simulink model "AN_Simulink_Model_v1_fil"  (R2019b)
settings: Solver=VariableStepAuto  StartTime=0.0  StopTime=testtime  RelTol=1e-3
InitFcn:
  | AN_InitFcn_Callback
StopFcn:
  | AN_StopFcn_Callback
undefined symbols (not defined in the file or in its folder): tdres
libraries: hdlmdlgenlib x193, simulink x4, fillib x1, dspsrcs4 x1
(part 5 of 6)

== system AN_Simulink_Model_v1_fil/Auditory Nerve Model/C2 Wideband Filter/Calculate C2filterout/Abs ==
  In1 : Inport
  Abs : Abs  SampleTime=2.08333333333333e-05  OutDataTypeStr=single
  Out1 : Outport
  wires:
  Abs/1 -> Out1/1
  In1/1 -> Abs/1

== system AN_Simulink_Model_v1_fil/Auditory Nerve Model/C2 Wideband Filter/Calculate C2filterout/Divide ==
  In1 : Inport
  In2 : Inport  Port=2
  Divide : Product  Inputs=*/  OutDataTypeStr=single  SampleTime=2.08333333333333e-05  SaturateOnIntegerOverflow=on  RndMeth=Zero
  Out1 : Outport
  wires:
  Divide/1 -> Out1/1
  In2/1 -> Divide/2
  In1/1 -> Divide/1

== system AN_Simulink_Model_v1_fil/Auditory Nerve Model/C2 Wideband Filter/Calculate C2filterout/Divide1 ==
  In1 : Inport
  In2 : Inport  Port=2
  Divide1 : Product  Inputs=*/  OutDataTypeStr=single  SampleTime=2.08333333333333e-05  SaturateOnIntegerOverflow=on  RndMeth=Zero
  Out1 : Outport
  wires:
  Divide1/1 -> Out1/1
  In2/1 -> Divide1/2
  In1/1 -> Divide1/1

== system AN_Simulink_Model_v1_fil/Auditory Nerve Model/C2 Wideband Filter/Calculate C2filterout/Product ==
  In1 : Inport
  In2 : Inport  Port=2
  Product : Product  Inputs=**  OutDataTypeStr=single  SampleTime=2.08333333333333e-05
  Out1 : Outport
  wires:
  Product/1 -> Out1/1
  In2/1 -> Product/2
  In1/1 -> Product/1

== system AN_Simulink_Model_v1_fil/Auditory Nerve Model/C2 Wideband Filter/Calculate C2filterout/Product1 ==
  In1 : Inport
  In2 : Inport  Port=2
  Product1 : Product  Inputs=**  OutDataTypeStr=single  SampleTime=2.08333333333333e-05
  Out1 : Outport
  wires:
  Product1/1 -> Out1/1
  In2/1 -> Product1/2
  In1/1 -> Product1/1

== system AN_Simulink_Model_v1_fil/Auditory Nerve Model/C2 Wideband Filter/Calculate C2filterout/Product2 ==
  In1 : Inport
  In2 : Inport  Port=2
  Product2 : Product  Inputs=**  OutDataTypeStr=single  SampleTime=2.08333333333333e-05
  Out1 : Outport
  wires:
  Product2/1 -> Out1/1
  In2/1 -> Product2/2
  In1/1 -> Product2/1

== system AN_Simulink_Model_v1_fil/Auditory Nerve Model/CP Wideband Gammatone Filter/Calculate wbout/Divide ==
  In1 : Inport
  In2 : Inport  Port=2
  Divide : Product  Inputs=*/  OutDataTypeStr=single  SampleTime=2.08333333333333e-05  SaturateOnIntegerOverflow=on  RndMeth=Zero
  Out1 : Outport
  wires:
  Divide/1 -> Out1/1
  In2/1 -> Divide/2
  In1/1 -> Divide/1

== system AN_Simulink_Model_v1_fil/Auditory Nerve Model/CP Wideband Gammatone Filter/Calculate wbout/Gain ==
  In1 : Inport
  In2 : Inport  Port=2
  Gain : Product  Inputs=**  OutDataTypeStr=single  SampleTime=2.08333333333333e-05
  Out1 : Outport
  wires:
  Gain/1 -> Out1/1
  In2/1 -> Gain/2
  In1/1 -> Gain/1

== system AN_Simulink_Model_v1_fil/Auditory Nerve Model/CP Wideband Gammatone Filter/Calculate wbout/MinMax_stage1_compare ==
  In1 : Inport
  In2 : Inport  Port=2
  MinMax_stage1_compare : RelationalOperator  Operator=<  OutDataTypeStr=boolean  SampleTime=2.08333333333333e-05  RndMeth=Nearest  InputSameDT=on
  Out1 : Outport
  wires:
  MinMax_stage1_compare/1 -> Out1/1
  In2/1 -> MinMax_stage1_compare/2
  In1/1 -> MinMax_stage1_compare/1

== system AN_Simulink_Model_v1_fil/Auditory Nerve Model/CP Wideband Gammatone Filter/Calculate wbout/Pow ==
  In1 : Inport
  In2 : Inport  Port=2
  Pow : Math  Operator=pow  SampleTime=2.08333333333333e-05  SaturateOnIntegerOverflow=on
  Out1 : Outport
  wires:
  Pow/1 -> Out1/1
  In2/1 -> Pow/2
  In1/1 -> Pow/1

== system AN_Simulink_Model_v1_fil/Auditory Nerve Model/CP Wideband Gammatone Filter/Calculate wbout/Product ==
  In1 : Inport
  In2 : Inport  Port=2
  Product : Product  Inputs=**  OutDataTypeStr=single  SampleTime=2.08333333333333e-05
  Out1 : Outport
  wires:
  Product/1 -> Out1/1
  In2/1 -> Product/2
  In1/1 -> Product/1

== system AN_Simulink_Model_v1_fil/Auditory Nerve Model/CP Wideband Gammatone Filter/Calculate wbout/Product1 ==
  In1 : Inport
  In2 : Inport  Port=2
  Product1 : Product  Inputs=**  OutDataTypeStr=single  SampleTime=2.08333333333333e-05
  Out1 : Outport
  wires:
  Product1/1 -> Out1/1
  In2/1 -> Product1/2
  In1/1 -> Product1/1

== system AN_Simulink_Model_v1_fil/Auditory Nerve Model/CP Wideband Gammatone Filter/MATLAB Function1/adder ==
  In1 : Inport
  In2 : Inport  Port=2
  adder : Sum  OutDataTypeStr=single  SampleTime=2.08333333333333e-05  SaturateOnIntegerOverflow=on  InputSameDT=on
  Out1 : Outport
  wires:
  adder/1 -> Out1/1
  In2/1 -> adder/2
  In1/1 -> adder/1

== system AN_Simulink_Model_v1_fil/Auditory Nerve Model/CP Wideband Gammatone Filter/MATLAB Function1/relop ==
  In1 : Inport
  In2 : Inport  Port=2
  relop : RelationalOperator  Operator=<=  OutDataTypeStr=boolean  SampleTime=2.08333333333333e-05  RndMeth=Nearest
  Out1 : Outport
  wires:
  relop/1 -> Out1/1
  In2/1 -> relop/2
  In1/1 -> relop/1

== system AN_Simulink_Model_v1_fil/Auditory Nerve Model/CP Wideband Gammatone Filter/MATLAB Function1/subtract ==
  In1 : Inport
  In2 : Inport  Port=2
  subtract : Sum  Inputs=+-  OutDataTypeStr=single  SampleTime=2.08333333333333e-05  SaturateOnIntegerOverflow=on  InputSameDT=on
  Out1 : Outport
  wires:
  subtract/1 -> Out1/1
  In2/1 -> subtract/2
  In1/1 -> subtract/1

== system AN_Simulink_Model_v1_fil/Auditory Nerve Model/CP Wideband Gammatone Filter/Third Order IIR Filter/Add ==
  In1 : Inport
  In2 : Inport  Port=2
  Add : Sum  OutDataTypeStr=single  SampleTime=2.08333333333333e-05  SaturateOnIntegerOverflow=on  InputSameDT=on
  Out1 : Outport
  wires:
  Add/1 -> Out1/1
  In2/1 -> Add/2
  In1/1 -> Add/1

== system AN_Simulink_Model_v1_fil/Auditory Nerve Model/CP Wideband Gammatone Filter/Third Order IIR Filter/Divide ==
  In1 : Inport
  In2 : Inport  Port=2
  Divide : Product  Inputs=*/  OutDataTypeStr=single  SampleTime=2.08333333333333e-05  SaturateOnIntegerOverflow=on  RndMeth=Zero
  Out1 : Outport
  wires:
  Divide/1 -> Out1/1
  In2/1 -> Divide/2
  In1/1 -> Divide/1

== system AN_Simulink_Model_v1_fil/Auditory Nerve Model/CP Wideband Gammatone Filter/Third Order IIR Filter/Divide1 ==
  In1 : Inport
  In2 : Inport  Port=2
  Divide1 : Product  Inputs=*/  OutDataTypeStr=single  SampleTime=2.08333333333333e-05  SaturateOnIntegerOverflow=on  RndMeth=Zero
  Out1 : Outport
  wires:
  Divide1/1 -> Out1/1
  In2/1 -> Divide1/2
  In1/1 -> Divide1/1

== system AN_Simulink_Model_v1_fil/Auditory Nerve Model/CP Wideband Gammatone Filter/Third Order IIR Filter/Divide2 ==
  In1 : Inport
  In2 : Inport  Port=2
  Divide2 : Product  Inputs=*/  OutDataTypeStr=single  SampleTime=2.08333333333333e-05  SaturateOnIntegerOverflow=on  RndMeth=Zero
  Out1 : Outport
  wires:
  Divide2/1 -> Out1/1
  In2/1 -> Divide2/2
  In1/1 -> Divide2/1

== system AN_Simulink_Model_v1_fil/Auditory Nerve Model/CP Wideband Gammatone Filter/Third Order IIR Filter/Product2 ==
  In1 : Inport
  In2 : Inport  Port=2
  Product2 : Product  Inputs=**  OutDataTypeStr=single  SampleTime=2.08333333333333e-05
  Out1 : Outport
  wires:
  Product2/1 -> Out1/1
  In2/1 -> Product2/2
  In1/1 -> Product2/1

== system AN_Simulink_Model_v1_fil/Auditory Nerve Model/CP Wideband Gammatone Filter/Third Order IIR Filter/Product21 ==
  In1 : Inport
  In2 : Inport  Port=2
  Product21 : Product  Inputs=**  OutDataTypeStr=single  SampleTime=2.08333333333333e-05
  Out1 : Outport
  wires:
  Product21/1 -> Out1/1
  In2/1 -> Product21/2
  In1/1 -> Product21/1

== system AN_Simulink_Model_v1_fil/Auditory Nerve Model/CP Wideband Gammatone Filter/Third Order IIR Filter/Product3_to_gain ==
  In1 : Inport
  Product3_to_gain : Gain  Gain=single(2)
  Out1 : Outport
  wires:
  Product3_to_gain/1 -> Out1/1
  In1/1 -> Product3_to_gain/1

== system AN_Simulink_Model_v1_fil/Auditory Nerve Model/CP Wideband Gammatone Filter/Third Order IIR Filter/Product4 ==
  In1 : Inport
  In2 : Inport  Port=2
  Product4 : Product  Inputs=**  OutDataTypeStr=single  SampleTime=2.08333333333333e-05
  Out1 : Outport
  wires:
  Product4/1 -> Out1/1
  In2/1 -> Product4/2
  In1/1 -> Product4/1

== system AN_Simulink_Model_v1_fil/Auditory Nerve Model/CP Wideband Gammatone Filter/Third Order IIR Filter/Product41 ==
  In1 : Inport
  In2 : Inport  Port=2
  Product41 : Product  Inputs=**  OutDataTypeStr=single  SampleTime=2.08333333333333e-05
  Out1 : Outport
  wires:
  Product41/1 -> Out1/1
  In2/1 -> Product41/2
  In1/1 -> Product41/1

== system AN_Simulink_Model_v1_fil/Auditory Nerve Model/CP Wideband Gammatone Filter/Third Order IIR Filter/Product5 ==
  In1 : Inport
  In2 : Inport  Port=2
  Product5 : Product  Inputs=**  OutDataTypeStr=single  SampleTime=2.08333333333333e-05
  Out1 : Outport
  wires:
  Product5/1 -> Out1/1
  In2/1 -> Product5/2
  In1/1 -> Product5/1

== system AN_Simulink_Model_v1_fil/Auditory Nerve Model/CP Wideband Gammatone Filter/Third Order IIR Filter/Product6 ==
  In1 : Inport
  In2 : Inport  Port=2
  Product6 : Product  Inputs=**  OutDataTypeStr=single  SampleTime=2.08333333333333e-05
  Out1 : Outport
  wires:
  Product6/1 -> Out1/1
  In2/1 -> Product6/2
  In1/1 -> Product6/1

== system AN_Simulink_Model_v1_fil/Auditory Nerve Model/CP Wideband Gammatone Filter/Third Order IIR Filter/Product61 ==
  In1 : Inport
  In2 : Inport  Port=2
  Product61 : Product  Inputs=**  OutDataTypeStr=single  SampleTime=2.08333333333333e-05
  Out1 : Outport
  wires:
  Product61/1 -> Out1/1
  In2/1 -> Product61/2
  In1/1 -> Product61/1

== system AN_Simulink_Model_v1_fil/Auditory Nerve Model/CP Wideband Gammatone Filter/Third Order IIR Filter/Product7 ==
  In1 : Inport
  In2 : Inport  Port=2
  Product7 : Product  Inputs=**  OutDataTypeStr=single  SampleTime=2.08333333333333e-05
  Out1 : Outport
  wires:
  Product7/1 -> Out1/1
  In2/1 -> Product7/2
  In1/1 -> Product7/1

== system AN_Simulink_Model_v1_fil/Auditory Nerve Model/CP Wideband Gammatone Filter/Third Order IIR Filter/Product71 ==
  In1 : Inport
  In2 : Inport  Port=2
  Product71 : Product  Inputs=**  OutDataTypeStr=single  SampleTime=2.08333333333333e-05
  Out1 : Outport
  wires:
  Product71/1 -> Out1/1
  In2/1 -> Product71/2
  In1/1 -> Product71/1

== system AN_Simulink_Model_v1_fil/Auditory Nerve Model/CP Wideband Gammatone Filter/Third Order IIR Filter/Product8 ==
  In1 : Inport
  In2 : Inport  Port=2
  Product8 : Product  Inputs=**  OutDataTypeStr=single  SampleTime=2.08333333333333e-05
  Out1 : Outport
  wires:
  Product8/1 -> Out1/1
  In2/1 -> Product8/2
  In1/1 -> Product8/1

== system AN_Simulink_Model_v1_fil/Auditory Nerve Model/CP Wideband Gammatone Filter/Third Order IIR Filter/Product81 ==
  In1 : Inport
  In2 : Inport  Port=2
  Product81 : Product  Inputs=**  OutDataTypeStr=single  SampleTime=2.08333333333333e-05
  Out1 : Outport
  wires:
  Product81/1 -> Out1/1
  In2/1 -> Product81/2
  In1/1 -> Product81/1

== system AN_Simulink_Model_v1_fil/Auditory Nerve Model/CP Wideband Gammatone Filter/Third Order IIR Filter/Product9 ==
  In1 : Inport
  In2 : Inport  Port=2
  Product9 : Product  Inputs=**  OutDataTypeStr=single  SampleTime=2.08333333333333e-05
  Out1 : Outport
  wires:
  Product9/1 -> Out1/1
  In2/1 -> Product9/2
  In1/1 -> Product9/1

== system AN_Simulink_Model_v1_fil/Auditory Nerve Model/CP Wideband Gammatone Filter/Third Order IIR Filter/Product91 ==
  In1 : Inport
  In2 : Inport  Port=2
  Product91 : Product  Inputs=**  OutDataTypeStr=single  SampleTime=2.08333333333333e-05
  Out1 : Outport
  wires:
  Product91/1 -> Out1/1
  In2/1 -> Product91/2
  In1/1 -> Product91/1

== system AN_Simulink_Model_v1_fil/Auditory Nerve Model/CP Wideband Gammatone Filter/Third Order IIR Filter/Subtract ==
  In1 : Inport
  In2 : Inport  Port=2
  Subtract : Sum  Inputs=+-  OutDataTypeStr=single  SampleTime=2.08333333333333e-05  SaturateOnIntegerOverflow=on  InputSameDT=on
  Out1 : Outport
  wires:
  Subtract/1 -> Out1/1
  In2/1 -> Subtract/2
  In1/1 -> Subtract/1

== system AN_Simulink_Model_v1_fil/Auditory Nerve Model/CP Wideband Gammatone Filter/Third Order IIR Filter/Sum1 ==
  In1 : Inport
  In2 : Inport  Port=2
  Sum1 : Sum  OutDataTypeStr=single  SampleTime=2.08333333333333e-05  SaturateOnIntegerOverflow=on  InputSameDT=on
  Out1 : Outport
  wires:
  Sum1/1 -> Out1/1
  In2/1 -> Sum1/2
  In1/1 -> Sum1/1

== system AN_Simulink_Model_v1_fil/Auditory Nerve Model/CP Wideband Gammatone Filter/Third Order IIR Filter/Sum2 ==
  In1 : Inport
  In2 : Inport  Port=2
  Sum2 : Sum  OutDataTypeStr=single  SampleTime=2.08333333333333e-05  SaturateOnIntegerOverflow=on  InputSameDT=on
  Out1 : Outport
  wires:
  Sum2/1 -> Out1/1
  In2/1 -> Sum2/2
  In1/1 -> Sum2/1

== system AN_Simulink_Model_v1_fil/Auditory Nerve Model/CP Wideband Gammatone Filter/Third Order IIR Filter/Sum3 ==
  In1 : Inport
  In2 : Inport  Port=2
  Sum3 : Sum  OutDataTypeStr=single  SampleTime=2.08333333333333e-05  SaturateOnIntegerOverflow=on  InputSameDT=on
  Out1 : Outport
  wires:
  Sum3/1 -> Out1/1
  In2/1 -> Sum3/2
  In1/1 -> Sum3/1

== system AN_Simulink_Model_v1_fil/Auditory Nerve Model/CP Wideband Gammatone Filter/Third Order IIR Filter/Sum4 ==
  In1 : Inport
  In2 : Inport  Port=2
  Sum4 : Sum  OutDataTypeStr=single  SampleTime=2.08333333333333e-05  SaturateOnIntegerOverflow=on  InputSameDT=on
  Out1 : Outport
  wires:
  Sum4/1 -> Out1/1
  In2/1 -> Sum4/2
  In1/1 -> Sum4/1

== system AN_Simulink_Model_v1_fil/Auditory Nerve Model/CP Wideband Gammatone Filter/Third Order IIR Filter/Sum5 ==
  In1 : Inport
  In2 : Inport  Port=2
  Sum5 : Sum  OutDataTypeStr=single  SampleTime=2.08333333333333e-05  SaturateOnIntegerOverflow=on  InputSameDT=on
  Out1 : Outport
  wires:
  Sum5/1 -> Out1/1
  In2/1 -> Sum5/2
  In1/1 -> Sum5/1

== system AN_Simulink_Model_v1_fil/Auditory Nerve Model/CP Wideband Gammatone Filter/Third Order IIR Filter/Sum6 ==
  In1 : Inport
  In2 : Inport  Port=2
  Sum6 : Sum  OutDataTypeStr=single  SampleTime=2.08333333333333e-05  SaturateOnIntegerOverflow=on  InputSameDT=on
  Out1 : Outport
  wires:
  Sum6/1 -> Out1/1
  In2/1 -> Sum6/2
  In1/1 -> Sum6/1

== system AN_Simulink_Model_v1_fil/Auditory Nerve Model/Subsystem/IHC C1 NL Logarithmic Function/Abs1 ==
  In1 : Inport
  Abs1 : Abs  SampleTime=2.08333333333333e-05  OutDataTypeStr=single
  Out1 : Outport
  wires:
  Abs1/1 -> Out1/1
  In1/1 -> Abs1/1

== system AN_Simulink_Model_v1_fil/Auditory Nerve Model/Subsystem/IHC C1 NL Logarithmic Function/Add1 ==
  In1 : Inport
  In2 : Inport  Port=2
  Add1 : Sum  OutDataTypeStr=single  SampleTime=2.08333333333333e-05  SaturateOnIntegerOverflow=on  InputSameDT=on
  Out1 : Outport
  wires:
  Add1/1 -> Out1/1
  In2/1 -> Add1/2
  In1/1 -> Add1/1

== system AN_Simulink_Model_v1_fil/Auditory Nerve Model/Subsystem/IHC C1 NL Logarithmic Function/Compare To Zero1_relop ==
  In1 : Inport
  In2 : Inport  Port=2
  Compare To Zero1_relop : RelationalOperator  Operator=<  OutDataTypeStr=boolean  SampleTime=2.08333333333333e-05  RndMeth=Nearest  InputSameDT=on
  Out1 : Outport
  wires:
  Compare To Zero1_relop/1 -> Out1/1
  In2/1 -> Compare To Zero1_relop/2
  In1/1 -> Compare To Zero1_relop/1

== system AN_Simulink_Model_v1_fil/Auditory Nerve Model/Subsystem/IHC C1 NL Logarithmic Function/Log1 ==
  In1 : Inport
  Log1 : Math  Operator=log  SampleTime=2.08333333333333e-05  SaturateOnIntegerOverflow=on
  Out1 : Outport
  wires:
  Log1/1 -> Out1/1
  In1/1 -> Log1/1

== system AN_Simulink_Model_v1_fil/Auditory Nerve Model/Subsystem/IHC C1 NL Logarithmic Function/Product3 ==
  In1 : Inport
  In2 : Inport  Port=2
  Product3 : Product  Inputs=**  OutDataTypeStr=single  SampleTime=2.08333333333333e-05
  Out1 : Outport
  wires:
  Product3/1 -> Out1/1
  In2/1 -> Product3/2
  In1/1 -> Product3/1

== system AN_Simulink_Model_v1_fil/Auditory Nerve Model/Subsystem/IHC C1 NL Logarithmic Function/Product4 ==
  In1 : Inport
  In2 : Inport  Port=2
  Product4 : Product  Inputs=**  OutDataTypeStr=single  SampleTime=2.08333333333333e-05
  Out1 : Outport
  wires:
  Product4/1 -> Out1/1
  In2/1 -> Product4/2
  In1/1 -> Product4/1

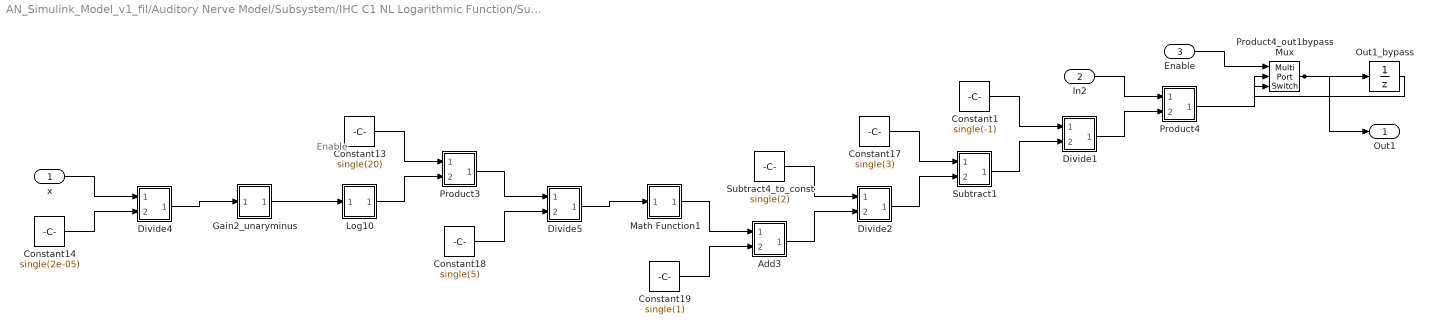
== system AN_Simulink_Model_v1_fil/Auditory Nerve Model/Subsystem/IHC C1 NL Logarithmic Function/Subsystem1 ==
  note: Enable
  x : Inport  OutDataTypeStr=single  PortDimensions=1  SampleTime=2.08333333333333e-05
  In2 : Inport  Port=2  OutDataTypeStr=single  PortDimensions=1  SampleTime=2.08333333333333e-05
  Enable : Inport  Port=3  OutDataTypeStr=boolean  SampleTime=2.08333333333333e-05
  Add3 : Subsystem
      mask Display: disp('NFP\nadd');
  Constant1 : Constant  Value=single(-1)  OutDataTypeStr=single  SampleTime=-1
  Constant13 : Constant  Value=single(20)  OutDataTypeStr=single  SampleTime=-1
  Constant14 : Constant  Value=single(2e-05)  OutDataTypeStr=single  SampleTime=-1
  Constant17 : Constant  Value=single(3)  OutDataTypeStr=single  SampleTime=-1
  Constant18 : Constant  Value=single(5)  OutDataTypeStr=single  SampleTime=-1
  Constant19 : Constant  Value=single(1)  OutDataTypeStr=single  SampleTime=-1
  Divide1 : Subsystem
      mask Display: disp('NFP\nmul');
  Divide2 : Subsystem
      mask Display: disp('NFP\nmul');
  Divide4 : Subsystem
      mask Display: disp('NFP\nmul');
  Divide5 : Subsystem
      mask Display: disp('NFP\nmul');
  Gain2_unaryminus : Subsystem
      mask Display: disp('NFP\numinus');
  Log10 : Subsystem
      mask Display: disp('NFP\nmath');
  Math Function1 : Subsystem
      mask Display: disp('NFP\nmath');
  Out1_bypass : UnitDelay  SampleTime=2.08333333333333e-05
  Product3 : Subsystem
      mask Display: disp('NFP\nmul');
  Product4 : Subsystem
      mask Display: disp('NFP\nmul');
  Product4_out1bypassMux : MultiPortSwitch  DataPortOrder=Zero-based contiguous  Inputs=2  zeroidx=on  OutDataTypeStr=single  SampleTime=2.08333333333333e-05
  Subtract1 : Subsystem
      mask Display: disp('NFP\nadd');
  Subtract4_to_const : Constant  Value=single(2)  OutDataTypeStr=single  SampleTime=-1
  Out1 : Outport  OutDataTypeStr=single  InitialOutput=0
  wires:
  Subtract1/1(Out1) -> Divide1/2(In2)
  Product4/1(Out1) -> Product4_out1bypassMux/3
  Product3/1(Out1) -> Divide5/1(In1)
  Math Function1/1(Out1) -> Add3/1(In1)
  Log10/1(Out1) -> Product3/2(In2)
  Divide5/1(Out1) -> Math Function1/1(In1)
  Divide4/1(Out1) -> Gain2_unaryminus/1(In1)
  Divide2/1(Out1) -> Subtract1/2(In2)
  Divide1/1(Out1) -> Product4/2(In2)
  Add3/1(Out1) -> Divide2/2(In2)
  Gain2_unaryminus/1(Out1) -> Log10/1(In1)
  Out1_bypass/1 -> Product4_out1bypassMux/2
  Product4_out1bypassMux/1 -> Out1/1, Out1_bypass/1
  Subtract4_to_const/1 -> Divide2/1(In1)
  Constant19/1 -> Add3/2(In2)
  Constant18/1 -> Divide5/2(In2)
  Constant17/1 -> Subtract1/1(In1)
  Constant14/1 -> Divide4/2(In2)
  Constant13/1 -> Product3/1(In1)
  Constant1/1 -> Divide1/1(In1)
  In2/1 -> Product4/1(In1)
  x/1 -> Divide4/1(In1)
  Enable/1 -> Product4_out1bypassMux/1

== system AN_Simulink_Model_v1_fil/Auditory Nerve Model/Subsystem/IHC C2 NL Logarithmic Function/Abs1 ==
  In1 : Inport
  Abs1 : Abs  SampleTime=2.08333333333333e-05  OutDataTypeStr=single
  Out1 : Outport
  wires:
  Abs1/1 -> Out1/1
  In1/1 -> Abs1/1

== system AN_Simulink_Model_v1_fil/Auditory Nerve Model/Subsystem/IHC C2 NL Logarithmic Function/Add1 ==
  In1 : Inport
  In2 : Inport  Port=2
  Add1 : Sum  OutDataTypeStr=single  SampleTime=2.08333333333333e-05  SaturateOnIntegerOverflow=on  InputSameDT=on
  Out1 : Outport
  wires:
  Add1/1 -> Out1/1
  In2/1 -> Add1/2
  In1/1 -> Add1/1

== system AN_Simulink_Model_v1_fil/Auditory Nerve Model/Subsystem/IHC C2 NL Logarithmic Function/Compare To Zero1_relop ==
  In1 : Inport
  In2 : Inport  Port=2
  Compare To Zero1_relop : RelationalOperator  Operator=<  OutDataTypeStr=boolean  SampleTime=2.08333333333333e-05  RndMeth=Nearest  InputSameDT=on
  Out1 : Outport
  wires:
  Compare To Zero1_relop/1 -> Out1/1
  In2/1 -> Compare To Zero1_relop/2
  In1/1 -> Compare To Zero1_relop/1

== system AN_Simulink_Model_v1_fil/Auditory Nerve Model/Subsystem/IHC C2 NL Logarithmic Function/Log1 ==
  In1 : Inport
  Log1 : Math  Operator=log  SampleTime=2.08333333333333e-05  SaturateOnIntegerOverflow=on
  Out1 : Outport
  wires:
  Log1/1 -> Out1/1
  In1/1 -> Log1/1

== system AN_Simulink_Model_v1_fil/Auditory Nerve Model/Subsystem/IHC C2 NL Logarithmic Function/Product3 ==
  In1 : Inport
  In2 : Inport  Port=2
  Product3 : Product  Inputs=**  OutDataTypeStr=single  SampleTime=2.08333333333333e-05
  Out1 : Outport
  wires:
  Product3/1 -> Out1/1
  In2/1 -> Product3/2
  In1/1 -> Product3/1

== system AN_Simulink_Model_v1_fil/Auditory Nerve Model/Subsystem/IHC C2 NL Logarithmic Function/Product4 ==
  In1 : Inport
  In2 : Inport  Port=2
  Product4 : Product  Inputs=**  OutDataTypeStr=single  SampleTime=2.08333333333333e-05
  Out1 : Outport
  wires:
  Product4/1 -> Out1/1
  In2/1 -> Product4/2
  In1/1 -> Product4/1

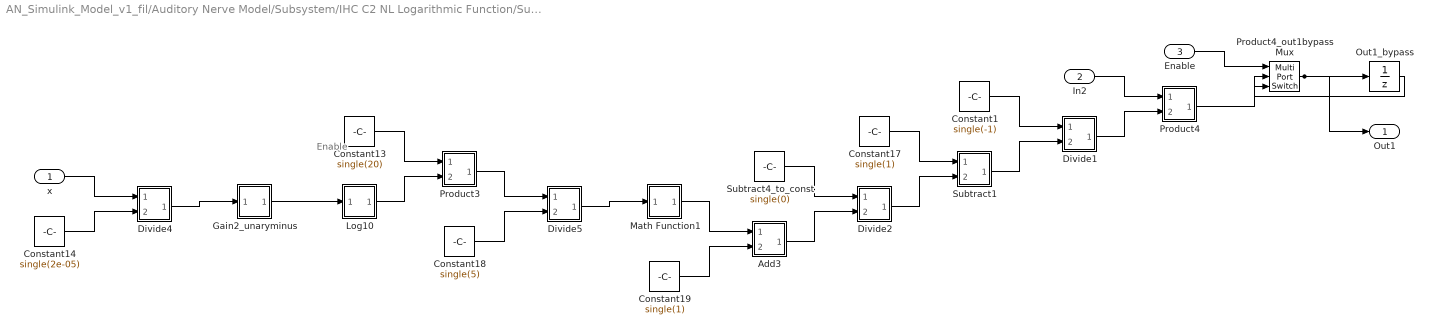
== system AN_Simulink_Model_v1_fil/Auditory Nerve Model/Subsystem/IHC C2 NL Logarithmic Function/Subsystem1 ==
  note: Enable
  x : Inport  OutDataTypeStr=single  PortDimensions=1  SampleTime=2.08333333333333e-05
  In2 : Inport  Port=2  OutDataTypeStr=single  PortDimensions=1  SampleTime=2.08333333333333e-05
  Enable : Inport  Port=3  OutDataTypeStr=boolean  SampleTime=2.08333333333333e-05
  Add3 : Subsystem
      mask Display: disp('NFP\nadd');
  Constant1 : Constant  Value=single(-1)  OutDataTypeStr=single  SampleTime=-1
  Constant13 : Constant  Value=single(20)  OutDataTypeStr=single  SampleTime=-1
  Constant14 : Constant  Value=single(2e-05)  OutDataTypeStr=single  SampleTime=-1
  Constant17 : Constant  Value=single(1)  OutDataTypeStr=single  SampleTime=-1
  Constant18 : Constant  Value=single(5)  OutDataTypeStr=single  SampleTime=-1
  Constant19 : Constant  Value=single(1)  OutDataTypeStr=single  SampleTime=-1
  Divide1 : Subsystem
      mask Display: disp('NFP\nmul');
  Divide2 : Subsystem
      mask Display: disp('NFP\nmul');
  Divide4 : Subsystem
      mask Display: disp('NFP\nmul');
  Divide5 : Subsystem
      mask Display: disp('NFP\nmul');
  Gain2_unaryminus : Subsystem
      mask Display: disp('NFP\numinus');
  Log10 : Subsystem
      mask Display: disp('NFP\nmath');
  Math Function1 : Subsystem
      mask Display: disp('NFP\nmath');
  Out1_bypass : UnitDelay  SampleTime=2.08333333333333e-05
  Product3 : Subsystem
      mask Display: disp('NFP\nmul');
  Product4 : Subsystem
      mask Display: disp('NFP\nmul');
  Product4_out1bypassMux : MultiPortSwitch  DataPortOrder=Zero-based contiguous  Inputs=2  zeroidx=on  OutDataTypeStr=single  SampleTime=2.08333333333333e-05
  Subtract1 : Subsystem
      mask Display: disp('NFP\nadd');
  Subtract4_to_const : Constant  Value=single(0)  OutDataTypeStr=single  SampleTime=-1
  Out1 : Outport  OutDataTypeStr=single  InitialOutput=0
  wires:
  Subtract1/1(Out1) -> Divide1/2(In2)
  Product4/1(Out1) -> Product4_out1bypassMux/3
  Product3/1(Out1) -> Divide5/1(In1)
  Math Function1/1(Out1) -> Add3/1(In1)
  Log10/1(Out1) -> Product3/2(In2)
  Divide5/1(Out1) -> Math Function1/1(In1)
  Divide4/1(Out1) -> Gain2_unaryminus/1(In1)
  Divide2/1(Out1) -> Subtract1/2(In2)
  Divide1/1(Out1) -> Product4/2(In2)
  Add3/1(Out1) -> Divide2/2(In2)
  Gain2_unaryminus/1(Out1) -> Log10/1(In1)
  Out1_bypass/1 -> Product4_out1bypassMux/2
  Product4_out1bypassMux/1 -> Out1/1, Out1_bypass/1
  Subtract4_to_const/1 -> Divide2/1(In1)
  Constant19/1 -> Add3/2(In2)
  Constant18/1 -> Divide5/2(In2)
  Constant17/1 -> Subtract1/1(In1)
  Constant14/1 -> Divide4/2(In2)
  Constant13/1 -> Product3/1(In1)
  Constant1/1 -> Divide1/1(In1)
  In2/1 -> Product4/1(In1)
  x/1 -> Divide4/1(In1)
  Enable/1 -> Product4_out1bypassMux/1

== system AN_Simulink_Model_v1_fil/Auditory Nerve Model/Subsystem/IHC LP Filter/Gain12_unaryminus ==
  In1 : Inport
  Gain12_unaryminus : UnaryMinus  SampleTime=2.08333333333333e-05
  Out1 : Outport
  wires:
  Gain12_unaryminus/1 -> Out1/1
  In1/1 -> Gain12_unaryminus/1

== system AN_Simulink_Model_v1_fil/Auditory Nerve Model/Subsystem/IHC LP Filter/Gain14_unaryminus ==
  In1 : Inport
  Gain14_unaryminus : UnaryMinus  SampleTime=2.08333333333333e-05
  Out1 : Outport
  wires:
  Gain14_unaryminus/1 -> Out1/1
  In1/1 -> Gain14_unaryminus/1

== system AN_Simulink_Model_v1_fil/Auditory Nerve Model/Subsystem/IHC LP Filter/Gain1_unaryminus ==
  In1 : Inport
  Gain1_unaryminus : UnaryMinus  SampleTime=2.08333333333333e-05
  Out1 : Outport
  wires:
  Gain1_unaryminus/1 -> Out1/1
  In1/1 -> Gain1_unaryminus/1

== system AN_Simulink_Model_v1_fil/Auditory Nerve Model/Subsystem/IHC LP Filter/Gain3_unaryminus ==
  In1 : Inport
  Gain3_unaryminus : UnaryMinus  SampleTime=2.08333333333333e-05
  Out1 : Outport
  wires:
  Gain3_unaryminus/1 -> Out1/1
  In1/1 -> Gain3_unaryminus/1

== system AN_Simulink_Model_v1_fil/Auditory Nerve Model/Subsystem/IHC LP Filter/Gain4_unaryminus ==
  In1 : Inport
  Gain4_unaryminus : UnaryMinus  SampleTime=2.08333333333333e-05
  Out1 : Outport
  wires:
  Gain4_unaryminus/1 -> Out1/1
  In1/1 -> Gain4_unaryminus/1

== system AN_Simulink_Model_v1_fil/Auditory Nerve Model/Subsystem/IHC LP Filter/Gain6_unaryminus ==
  In1 : Inport
  Gain6_unaryminus : UnaryMinus  SampleTime=2.08333333333333e-05
  Out1 : Outport
  wires:
  Gain6_unaryminus/1 -> Out1/1
  In1/1 -> Gain6_unaryminus/1

== system AN_Simulink_Model_v1_fil/Auditory Nerve Model/Subsystem/IHC LP Filter/Gain9_unaryminus ==
  In1 : Inport
  Gain9_unaryminus : UnaryMinus  SampleTime=2.08333333333333e-05
  Out1 : Outport
  wires:
  Gain9_unaryminus/1 -> Out1/1
  In1/1 -> Gain9_unaryminus/1

== system AN_Simulink_Model_v1_fil/Auditory Nerve Model/Subsystem/IHC LP Filter/Product12 ==
  In1 : Inport
  In2 : Inport  Port=2
  Product12 : Product  Inputs=**  OutDataTypeStr=single  SampleTime=2.08333333333333e-05
  Out1 : Outport
  wires:
  Product12/1 -> Out1/1
  In2/1 -> Product12/2
  In1/1 -> Product12/1

== system AN_Simulink_Model_v1_fil/Auditory Nerve Model/Subsystem/IHC LP Filter/Product13 ==
  In1 : Inport
  In2 : Inport  Port=2
  Product13 : Product  Inputs=**  OutDataTypeStr=single  SampleTime=2.08333333333333e-05
  Out1 : Outport
  wires:
  Product13/1 -> Out1/1
  In2/1 -> Product13/2
  In1/1 -> Product13/1

== system AN_Simulink_Model_v1_fil/Auditory Nerve Model/Subsystem/IHC LP Filter/Product14 ==
  In1 : Inport
  In2 : Inport  Port=2
  Product14 : Product  Inputs=**  OutDataTypeStr=single  SampleTime=2.08333333333333e-05
  Out1 : Outport
  wires:
  Product14/1 -> Out1/1
  In2/1 -> Product14/2
  In1/1 -> Product14/1

== system AN_Simulink_Model_v1_fil/Auditory Nerve Model/Subsystem/IHC LP Filter/Product17 ==
  In1 : Inport
  In2 : Inport  Port=2
  Product17 : Product  Inputs=**  OutDataTypeStr=single  SampleTime=2.08333333333333e-05
  Out1 : Outport
  wires:
  Product17/1 -> Out1/1
  In2/1 -> Product17/2
  In1/1 -> Product17/1

== system AN_Simulink_Model_v1_fil/Auditory Nerve Model/Subsystem/IHC LP Filter/Product18 ==
  In1 : Inport
  In2 : Inport  Port=2
  Product18 : Product  Inputs=**  OutDataTypeStr=single  SampleTime=2.08333333333333e-05
  Out1 : Outport
  wires:
  Product18/1 -> Out1/1
  In2/1 -> Product18/2
  In1/1 -> Product18/1

== system AN_Simulink_Model_v1_fil/Auditory Nerve Model/Subsystem/IHC LP Filter/Product19 ==
  In1 : Inport
  In2 : Inport  Port=2
  Product19 : Product  Inputs=**  OutDataTypeStr=single  SampleTime=2.08333333333333e-05
  Out1 : Outport
  wires:
  Product19/1 -> Out1/1
  In2/1 -> Product19/2
  In1/1 -> Product19/1

== system AN_Simulink_Model_v1_fil/Auditory Nerve Model/Subsystem/IHC LP Filter/Product2 ==
  In1 : Inport
  In2 : Inport  Port=2
  Product2 : Product  Inputs=**  OutDataTypeStr=single  SampleTime=2.08333333333333e-05
  Out1 : Outport
  wires:
  Product2/1 -> Out1/1
  In2/1 -> Product2/2
  In1/1 -> Product2/1

== system AN_Simulink_Model_v1_fil/Auditory Nerve Model/Subsystem/IHC LP Filter/Product22 ==
  In1 : Inport
  In2 : Inport  Port=2
  Product22 : Product  Inputs=**  OutDataTypeStr=single  SampleTime=2.08333333333333e-05
  Out1 : Outport
  wires:
  Product22/1 -> Out1/1
  In2/1 -> Product22/2
  In1/1 -> Product22/1

== system AN_Simulink_Model_v1_fil/Auditory Nerve Model/Subsystem/IHC LP Filter/Product23 ==
  In1 : Inport
  In2 : Inport  Port=2
  Product23 : Product  Inputs=**  OutDataTypeStr=single  SampleTime=2.08333333333333e-05
  Out1 : Outport
  wires:
  Product23/1 -> Out1/1
  In2/1 -> Product23/2
  In1/1 -> Product23/1

== system AN_Simulink_Model_v1_fil/Auditory Nerve Model/Subsystem/IHC LP Filter/Product24 ==
  In1 : Inport
  In2 : Inport  Port=2
  Product24 : Product  Inputs=**  OutDataTypeStr=single  SampleTime=2.08333333333333e-05
  Out1 : Outport
  wires:
  Product24/1 -> Out1/1
  In2/1 -> Product24/2
  In1/1 -> Product24/1

== system AN_Simulink_Model_v1_fil/Auditory Nerve Model/Subsystem/IHC LP Filter/Product27 ==
  In1 : Inport
  In2 : Inport  Port=2
  Product27 : Product  Inputs=**  OutDataTypeStr=single  SampleTime=2.08333333333333e-05
  Out1 : Outport
  wires:
  Product27/1 -> Out1/1
  In2/1 -> Product27/2
  In1/1 -> Product27/1

== system AN_Simulink_Model_v1_fil/Auditory Nerve Model/Subsystem/IHC LP Filter/Product28 ==
  In1 : Inport
  In2 : Inport  Port=2
  Product28 : Product  Inputs=**  OutDataTypeStr=single  SampleTime=2.08333333333333e-05
  Out1 : Outport
  wires:
  Product28/1 -> Out1/1
  In2/1 -> Product28/2
  In1/1 -> Product28/1

== system AN_Simulink_Model_v1_fil/Auditory Nerve Model/Subsystem/IHC LP Filter/Product29 ==
  In1 : Inport
  In2 : Inport  Port=2
  Product29 : Product  Inputs=**  OutDataTypeStr=single  SampleTime=2.08333333333333e-05
  Out1 : Outport
  wires:
  Product29/1 -> Out1/1
  In2/1 -> Product29/2
  In1/1 -> Product29/1

== system AN_Simulink_Model_v1_fil/Auditory Nerve Model/Subsystem/IHC LP Filter/Product3 ==
  In1 : Inport
  In2 : Inport  Port=2
  Product3 : Product  Inputs=**  OutDataTypeStr=single  SampleTime=2.08333333333333e-05
  Out1 : Outport
  wires:
  Product3/1 -> Out1/1
  In2/1 -> Product3/2
  In1/1 -> Product3/1

== system AN_Simulink_Model_v1_fil/Auditory Nerve Model/Subsystem/IHC LP Filter/Product32 ==
  In1 : Inport
  In2 : Inport  Port=2
  Product32 : Product  Inputs=**  OutDataTypeStr=single  SampleTime=2.08333333333333e-05
  Out1 : Outport
  wires:
  Product32/1 -> Out1/1
  In2/1 -> Product32/2
  In1/1 -> Product32/1

== system AN_Simulink_Model_v1_fil/Auditory Nerve Model/Subsystem/IHC LP Filter/Product33 ==
  In1 : Inport
  In2 : Inport  Port=2
  Product33 : Product  Inputs=**  OutDataTypeStr=single  SampleTime=2.08333333333333e-05
  Out1 : Outport
  wires:
  Product33/1 -> Out1/1
  In2/1 -> Product33/2
  In1/1 -> Product33/1

== system AN_Simulink_Model_v1_fil/Auditory Nerve Model/Subsystem/IHC LP Filter/Product34 ==
  In1 : Inport
  In2 : Inport  Port=2
  Product34 : Product  Inputs=**  OutDataTypeStr=single  SampleTime=2.08333333333333e-05
  Out1 : Outport
  wires:
  Product34/1 -> Out1/1
  In2/1 -> Product34/2
  In1/1 -> Product34/1

== system AN_Simulink_Model_v1_fil/Auditory Nerve Model/Subsystem/IHC LP Filter/Product4 ==
  In1 : Inport
  In2 : Inport  Port=2
  Product4 : Product  Inputs=**  OutDataTypeStr=single  SampleTime=2.08333333333333e-05
  Out1 : Outport
  wires:
  Product4/1 -> Out1/1
  In2/1 -> Product4/2
  In1/1 -> Product4/1

== system AN_Simulink_Model_v1_fil/Auditory Nerve Model/Subsystem/IHC LP Filter/Product7 ==
  In1 : Inport
  In2 : Inport  Port=2
  Product7 : Product  Inputs=**  OutDataTypeStr=single  SampleTime=2.08333333333333e-05
  Out1 : Outport
  wires:
  Product7/1 -> Out1/1
  In2/1 -> Product7/2
  In1/1 -> Product7/1

== system AN_Simulink_Model_v1_fil/Auditory Nerve Model/Subsystem/IHC LP Filter/Product8 ==
  In1 : Inport
  In2 : Inport  Port=2
  Product8 : Product  Inputs=**  OutDataTypeStr=single  SampleTime=2.08333333333333e-05
  Out1 : Outport
  wires:
  Product8/1 -> Out1/1
  In2/1 -> Product8/2
  In1/1 -> Product8/1

== system AN_Simulink_Model_v1_fil/Auditory Nerve Model/Subsystem/IHC LP Filter/Product9 ==
  In1 : Inport
  In2 : Inport  Port=2
  Product9 : Product  Inputs=**  OutDataTypeStr=single  SampleTime=2.08333333333333e-05
  Out1 : Outport
  wires:
  Product9/1 -> Out1/1
  In2/1 -> Product9/2
  In1/1 -> Product9/1

== system AN_Simulink_Model_v1_fil/Auditory Nerve Model/Subsystem/IHC LP Filter/Sum10 ==
  In1 : Inport
  In2 : Inport  Port=2
  Sum10 : Sum  OutDataTypeStr=single  SampleTime=2.08333333333333e-05  SaturateOnIntegerOverflow=on  InputSameDT=on
  Out1 : Outport
  wires:
  Sum10/1 -> Out1/1
  In2/1 -> Sum10/2
  In1/1 -> Sum10/1

== system AN_Simulink_Model_v1_fil/Auditory Nerve Model/Subsystem/IHC LP Filter/Sum11 ==
  In1 : Inport
  In2 : Inport  Port=2
  Sum11 : Sum  OutDataTypeStr=single  SampleTime=2.08333333333333e-05  SaturateOnIntegerOverflow=on  InputSameDT=on
  Out1 : Outport
  wires:
  Sum11/1 -> Out1/1
  In2/1 -> Sum11/2
  In1/1 -> Sum11/1

== system AN_Simulink_Model_v1_fil/Auditory Nerve Model/Subsystem/IHC LP Filter/Sum12 ==
  In1 : Inport
  In2 : Inport  Port=2
  Sum12 : Sum  OutDataTypeStr=single  SampleTime=2.08333333333333e-05  SaturateOnIntegerOverflow=on  InputSameDT=on
  Out1 : Outport
  wires:
  Sum12/1 -> Out1/1
  In2/1 -> Sum12/2
  In1/1 -> Sum12/1

== system AN_Simulink_Model_v1_fil/Auditory Nerve Model/Subsystem/IHC LP Filter/Sum13 ==
  In1 : Inport
  In2 : Inport  Port=2
  Sum13 : Sum  OutDataTypeStr=single  SampleTime=2.08333333333333e-05  SaturateOnIntegerOverflow=on  InputSameDT=on
  Out1 : Outport
  wires:
  Sum13/1 -> Out1/1
  In2/1 -> Sum13/2
  In1/1 -> Sum13/1

== system AN_Simulink_Model_v1_fil/Auditory Nerve Model/Subsystem/IHC LP Filter/Sum16 ==
  In1 : Inport
  In2 : Inport  Port=2
  Sum16 : Sum  OutDataTypeStr=single  SampleTime=2.08333333333333e-05  SaturateOnIntegerOverflow=on  InputSameDT=on
  Out1 : Outport
  wires:
  Sum16/1 -> Out1/1
  In2/1 -> Sum16/2
  In1/1 -> Sum16/1

== system AN_Simulink_Model_v1_fil/Auditory Nerve Model/Subsystem/IHC LP Filter/Sum17 ==
  In1 : Inport
  In2 : Inport  Port=2
  Sum17 : Sum  OutDataTypeStr=single  SampleTime=2.08333333333333e-05  SaturateOnIntegerOverflow=on  InputSameDT=on
  Out1 : Outport
  wires:
  Sum17/1 -> Out1/1
  In2/1 -> Sum17/2
  In1/1 -> Sum17/1

== system AN_Simulink_Model_v1_fil/Auditory Nerve Model/Subsystem/IHC LP Filter/Sum2 ==
  In1 : Inport
  In2 : Inport  Port=2
  Sum2 : Sum  OutDataTypeStr=single  SampleTime=2.08333333333333e-05  SaturateOnIntegerOverflow=on  InputSameDT=on
  Out1 : Outport
  wires:
  Sum2/1 -> Out1/1
  In2/1 -> Sum2/2
  In1/1 -> Sum2/1

== system AN_Simulink_Model_v1_fil/Auditory Nerve Model/Subsystem/IHC LP Filter/Sum20 ==
  In1 : Inport
  In2 : Inport  Port=2
  Sum20 : Sum  OutDataTypeStr=single  SampleTime=2.08333333333333e-05  SaturateOnIntegerOverflow=on  InputSameDT=on
  Out1 : Outport
  wires:
  Sum20/1 -> Out1/1
  In2/1 -> Sum20/2
  In1/1 -> Sum20/1

== system AN_Simulink_Model_v1_fil/Auditory Nerve Model/Subsystem/IHC LP Filter/Sum21 ==
  In1 : Inport
  In2 : Inport  Port=2
  Sum21 : Sum  OutDataTypeStr=single  SampleTime=2.08333333333333e-05  SaturateOnIntegerOverflow=on  InputSameDT=on
  Out1 : Outport
  wires:
  Sum21/1 -> Out1/1
  In2/1 -> Sum21/2
  In1/1 -> Sum21/1

== system AN_Simulink_Model_v1_fil/Auditory Nerve Model/Subsystem/IHC LP Filter/Sum24 ==
  In1 : Inport
  In2 : Inport  Port=2
  Sum24 : Sum  OutDataTypeStr=single  SampleTime=2.08333333333333e-05  SaturateOnIntegerOverflow=on  InputSameDT=on
  Out1 : Outport
  wires:
  Sum24/1 -> Out1/1
  In2/1 -> Sum24/2
  In1/1 -> Sum24/1

== system AN_Simulink_Model_v1_fil/Auditory Nerve Model/Subsystem/IHC LP Filter/Sum25 ==
  In1 : Inport
  In2 : Inport  Port=2
  Sum25 : Sum  OutDataTypeStr=single  SampleTime=2.08333333333333e-05  SaturateOnIntegerOverflow=on  InputSameDT=on
  Out1 : Outport
  wires:
  Sum25/1 -> Out1/1
  In2/1 -> Sum25/2
  In1/1 -> Sum25/1

== system AN_Simulink_Model_v1_fil/Auditory Nerve Model/Subsystem/IHC LP Filter/Sum3 ==
  In1 : Inport
  In2 : Inport  Port=2
  Sum3 : Sum  OutDataTypeStr=single  SampleTime=2.08333333333333e-05  SaturateOnIntegerOverflow=on  InputSameDT=on
  Out1 : Outport
  wires:
  Sum3/1 -> Out1/1
  In2/1 -> Sum3/2
  In1/1 -> Sum3/1

== system AN_Simulink_Model_v1_fil/Auditory Nerve Model/Subsystem/IHC LP Filter/Sum6 ==
  In1 : Inport
  In2 : Inport  Port=2
  Sum6 : Sum  OutDataTypeStr=single  SampleTime=2.08333333333333e-05  SaturateOnIntegerOverflow=on  InputSameDT=on
  Out1 : Outport
  wires:
  Sum6/1 -> Out1/1
  In2/1 -> Sum6/2
  In1/1 -> Sum6/1

== system AN_Simulink_Model_v1_fil/Auditory Nerve Model/Subsystem/IHC LP Filter/Sum7 ==
  In1 : Inport
  In2 : Inport  Port=2
  Sum7 : Sum  OutDataTypeStr=single  SampleTime=2.08333333333333e-05  SaturateOnIntegerOverflow=on  InputSameDT=on
  Out1 : Outport
  wires:
  Sum7/1 -> Out1/1
  In2/1 -> Sum7/2
  In1/1 -> Sum7/1

== system AN_Simulink_Model_v1_fil/Auditory Nerve Model/Subsystem1/Calculate tauc1/Add ==
  In1 : Inport
  In2 : Inport  Port=2
  Add : Sum  OutDataTypeStr=single  SampleTime=2.08333333333333e-05  SaturateOnIntegerOverflow=on  InputSameDT=on
  Out1 : Outport
  wires:
  Add/1 -> Out1/1
  In2/1 -> Add/2
  In1/1 -> Add/1

== system AN_Simulink_Model_v1_fil/Auditory Nerve Model/Subsystem1/Calculate tauc1/Product_to_gain ==
  In1 : Inport
  Product_to_gain : Gain  Gain=single(1)
  Out1 : Outport
  wires:
  Product_to_gain/1 -> Out1/1
  In1/1 -> Product_to_gain/1

== system AN_Simulink_Model_v1_fil/Auditory Nerve Model/Subsystem1/Calculate tauc1/Subtract ==
  In1 : Inport
  In2 : Inport  Port=2
  Subtract : Sum  Inputs=+-  OutDataTypeStr=single  SampleTime=2.08333333333333e-05  SaturateOnIntegerOverflow=on  InputSameDT=on
  Out1 : Outport
  wires:
  Subtract/1 -> Out1/1
  In2/1 -> Subtract/2
  In1/1 -> Subtract/1

== system AN_Simulink_Model_v1_fil/Auditory Nerve Model/Subsystem1/NL After OHC Function/Abs ==
  In1 : Inport
  Abs : Abs  SampleTime=2.08333333333333e-05  OutDataTypeStr=single
  Out1 : Outport
  wires:
  Abs/1 -> Out1/1
  In1/1 -> Abs/1

== system AN_Simulink_Model_v1_fil/Auditory Nerve Model/Subsystem1/NL After OHC Function/Add3 ==
  In1 : Inport
  In2 : Inport  Port=2
  Add3 : Sum  OutDataTypeStr=single  SampleTime=2.08333333333333e-05  SaturateOnIntegerOverflow=on  InputSameDT=on
  Out1 : Outport
  wires:
  Add3/1 -> Out1/1
  In2/1 -> Add3/2
  In1/1 -> Add3/1

== system AN_Simulink_Model_v1_fil/Auditory Nerve Model/Subsystem1/NL After OHC Function/Divide1 ==
  In1 : Inport
  In2 : Inport  Port=2
  Divide1 : Product  Inputs=*/  OutDataTypeStr=single  SampleTime=2.08333333333333e-05  SaturateOnIntegerOverflow=on  RndMeth=Zero
  Out1 : Outport
  wires:
  Divide1/1 -> Out1/1
  In2/1 -> Divide1/2
  In1/1 -> Divide1/1

== system AN_Simulink_Model_v1_fil/Auditory Nerve Model/Subsystem1/NL After OHC Function/Exp ==
  In1 : Inport
  Exp : Math  SampleTime=2.08333333333333e-05  SaturateOnIntegerOverflow=on
  Out1 : Outport
  wires:
  Exp/1 -> Out1/1
  In1/1 -> Exp/1

== system AN_Simulink_Model_v1_fil/Auditory Nerve Model/Subsystem1/NL After OHC Function/Gain2_unaryminus ==
  In1 : Inport
  Gain2_unaryminus : UnaryMinus  SampleTime=2.08333333333333e-05
  Out1 : Outport
  wires:
  Gain2_unaryminus/1 -> Out1/1
  In1/1 -> Gain2_unaryminus/1

== system AN_Simulink_Model_v1_fil/Auditory Nerve Model/Subsystem1/NL After OHC Function/Product3 ==
  In1 : Inport
  In2 : Inport  Port=2
  Product3 : Product  Inputs=**  OutDataTypeStr=single  SampleTime=2.08333333333333e-05
  Out1 : Outport
  wires:
  Product3/1 -> Out1/1
  In2/1 -> Product3/2
  In1/1 -> Product3/1

== system AN_Simulink_Model_v1_fil/Auditory Nerve Model/Subsystem1/NL After OHC Function/Product4 ==
  In1 : Inport
  In2 : Inport  Port=2
  Product4 : Product  Inputs=**  OutDataTypeStr=single  SampleTime=2.08333333333333e-05
  Out1 : Outport
  wires:
  Product4/1 -> Out1/1
  In2/1 -> Product4/2
  In1/1 -> Product4/1

== system AN_Simulink_Model_v1_fil/Auditory Nerve Model/Subsystem1/NL After OHC Function/Saturation_LowerRelop ==
  In1 : Inport
  In2 : Inport  Port=2
  Saturation_LowerRelop : RelationalOperator  Operator=>  OutDataTypeStr=boolean  SampleTime=2.08333333333333e-05  RndMeth=Nearest
  Out1 : Outport
  wires:
  Saturation_LowerRelop/1 -> Out1/1
  In2/1 -> Saturation_LowerRelop/2
  In1/1 -> Saturation_LowerRelop/1

== system AN_Simulink_Model_v1_fil/Auditory Nerve Model/Subsystem1/NL After OHC Function/Saturation_UpperRelop ==
  In1 : Inport
  In2 : Inport  Port=2
  Saturation_UpperRelop : RelationalOperator  Operator=<  OutDataTypeStr=boolean  SampleTime=2.08333333333333e-05  RndMeth=Nearest
  Out1 : Outport
  wires:
  Saturation_UpperRelop/1 -> Out1/1
  In2/1 -> Saturation_UpperRelop/2
  In1/1 -> Saturation_UpperRelop/1

== system AN_Simulink_Model_v1_fil/Auditory Nerve Model/Subsystem1/OHC LP Filter/Gain1_unaryminus ==
  In1 : Inport
  Gain1_unaryminus : UnaryMinus  SampleTime=2.08333333333333e-05
  Out1 : Outport
  wires:
  Gain1_unaryminus/1 -> Out1/1
  In1/1 -> Gain1_unaryminus/1

== system AN_Simulink_Model_v1_fil/Auditory Nerve Model/Subsystem1/OHC LP Filter/Gain2_unaryminus ==
  In1 : Inport
  Gain2_unaryminus : UnaryMinus  SampleTime=2.08333333333333e-05
  Out1 : Outport
  wires:
  Gain2_unaryminus/1 -> Out1/1
  In1/1 -> Gain2_unaryminus/1

== system AN_Simulink_Model_v1_fil/Auditory Nerve Model/Subsystem1/OHC LP Filter/Gain3_unaryminus ==
  In1 : Inport
  Gain3_unaryminus : UnaryMinus  SampleTime=2.08333333333333e-05
  Out1 : Outport
  wires:
  Gain3_unaryminus/1 -> Out1/1
  In1/1 -> Gain3_unaryminus/1

== system AN_Simulink_Model_v1_fil/Auditory Nerve Model/Subsystem1/OHC LP Filter/Gain5_unaryminus ==
  In1 : Inport
  Gain5_unaryminus : UnaryMinus  SampleTime=2.08333333333333e-05
  Out1 : Outport
  wires:
  Gain5_unaryminus/1 -> Out1/1
  In1/1 -> Gain5_unaryminus/1

== system AN_Simulink_Model_v1_fil/Auditory Nerve Model/Subsystem1/OHC LP Filter/Product ==
  In1 : Inport
  In2 : Inport  Port=2
  Product : Product  Inputs=**  OutDataTypeStr=single  SampleTime=2.08333333333333e-05
  Out1 : Outport
  wires:
  Product/1 -> Out1/1
  In2/1 -> Product/2
  In1/1 -> Product/1

== system AN_Simulink_Model_v1_fil/Auditory Nerve Model/Subsystem1/OHC LP Filter/Product1 ==
  In1 : Inport
  In2 : Inport  Port=2
  Product1 : Product  Inputs=**  OutDataTypeStr=single  SampleTime=2.08333333333333e-05
  Out1 : Outport
  wires:
  Product1/1 -> Out1/1
  In2/1 -> Product1/2
  In1/1 -> Product1/1

== system AN_Simulink_Model_v1_fil/Auditory Nerve Model/Subsystem1/OHC LP Filter/Product2 ==
  In1 : Inport
  In2 : Inport  Port=2
  Product2 : Product  Inputs=**  OutDataTypeStr=single  SampleTime=2.08333333333333e-05
  Out1 : Outport
  wires:
  Product2/1 -> Out1/1
  In2/1 -> Product2/2
  In1/1 -> Product2/1

== system AN_Simulink_Model_v1_fil/Auditory Nerve Model/Subsystem1/OHC LP Filter/Product3 ==
  In1 : Inport
  In2 : Inport  Port=2
  Product3 : Product  Inputs=**  OutDataTypeStr=single  SampleTime=2.08333333333333e-05
  Out1 : Outport
  wires:
  Product3/1 -> Out1/1
  In2/1 -> Product3/2
  In1/1 -> Product3/1

== system AN_Simulink_Model_v1_fil/Auditory Nerve Model/Subsystem1/OHC LP Filter/Product4 ==
  In1 : Inport
  In2 : Inport  Port=2
  Product4 : Product  Inputs=**  OutDataTypeStr=single  SampleTime=2.08333333333333e-05
  Out1 : Outport
  wires:
  Product4/1 -> Out1/1
  In2/1 -> Product4/2
  In1/1 -> Product4/1

== system AN_Simulink_Model_v1_fil/Auditory Nerve Model/Subsystem1/OHC LP Filter/Product5 ==
  In1 : Inport
  In2 : Inport  Port=2
  Product5 : Product  Inputs=**  OutDataTypeStr=single  SampleTime=2.08333333333333e-05
  Out1 : Outport
  wires:
  Product5/1 -> Out1/1
  In2/1 -> Product5/2
  In1/1 -> Product5/1

== system AN_Simulink_Model_v1_fil/Auditory Nerve Model/Subsystem1/OHC LP Filter/Product6 ==
  In1 : Inport
  In2 : Inport  Port=2
  Product6 : Product  Inputs=**  OutDataTypeStr=single  SampleTime=2.08333333333333e-05
  Out1 : Outport
  wires:
  Product6/1 -> Out1/1
  In2/1 -> Product6/2
  In1/1 -> Product6/1

== system AN_Simulink_Model_v1_fil/Auditory Nerve Model/Subsystem1/OHC LP Filter/Product7 ==
  In1 : Inport
  In2 : Inport  Port=2
  Product7 : Product  Inputs=**  OutDataTypeStr=single  SampleTime=2.08333333333333e-05
  Out1 : Outport
  wires:
  Product7/1 -> Out1/1
  In2/1 -> Product7/2
  In1/1 -> Product7/1

== system AN_Simulink_Model_v1_fil/Auditory Nerve Model/Subsystem1/OHC LP Filter/Product8 ==
  In1 : Inport
  In2 : Inport  Port=2
  Product8 : Product  Inputs=**  OutDataTypeStr=single  SampleTime=2.08333333333333e-05
  Out1 : Outport
  wires:
  Product8/1 -> Out1/1
  In2/1 -> Product8/2
  In1/1 -> Product8/1

== system AN_Simulink_Model_v1_fil/Auditory Nerve Model/Subsystem1/OHC LP Filter/Product9 ==
  In1 : Inport
  In2 : Inport  Port=2
  Product9 : Product  Inputs=**  OutDataTypeStr=single  SampleTime=2.08333333333333e-05
  Out1 : Outport
  wires:
  Product9/1 -> Out1/1
  In2/1 -> Product9/2
  In1/1 -> Product9/1

== system AN_Simulink_Model_v1_fil/Auditory Nerve Model/Subsystem1/OHC LP Filter/Sum ==
  In1 : Inport
  In2 : Inport  Port=2
  Sum : Sum  OutDataTypeStr=single  SampleTime=2.08333333333333e-05  SaturateOnIntegerOverflow=on  InputSameDT=on
  Out1 : Outport
  wires:
  Sum/1 -> Out1/1
  In2/1 -> Sum/2
  In1/1 -> Sum/1

== system AN_Simulink_Model_v1_fil/Auditory Nerve Model/Subsystem1/OHC LP Filter/Sum1 ==
  In1 : Inport
  In2 : Inport  Port=2
  Sum1 : Sum  OutDataTypeStr=single  SampleTime=2.08333333333333e-05  SaturateOnIntegerOverflow=on  InputSameDT=on
  Out1 : Outport
  wires:
  Sum1/1 -> Out1/1
  In2/1 -> Sum1/2
  In1/1 -> Sum1/1

== system AN_Simulink_Model_v1_fil/Auditory Nerve Model/Subsystem1/OHC LP Filter/Sum2 ==
  In1 : Inport
  In2 : Inport  Port=2
  Sum2 : Sum  OutDataTypeStr=single  SampleTime=2.08333333333333e-05  SaturateOnIntegerOverflow=on  InputSameDT=on
  Out1 : Outport
  wires:
  Sum2/1 -> Out1/1
  In2/1 -> Sum2/2
  In1/1 -> Sum2/1

== system AN_Simulink_Model_v1_fil/Auditory Nerve Model/Subsystem1/OHC LP Filter/Sum3 ==
  In1 : Inport
  In2 : Inport  Port=2
  Sum3 : Sum  OutDataTypeStr=single  SampleTime=2.08333333333333e-05  SaturateOnIntegerOverflow=on  InputSameDT=on
  Out1 : Outport
  wires:
  Sum3/1 -> Out1/1
  In2/1 -> Sum3/2
  In1/1 -> Sum3/1

== system AN_Simulink_Model_v1_fil/Auditory Nerve Model/Subsystem1/OHC LP Filter/Sum4 ==
  In1 : Inport
  In2 : Inport  Port=2
  Sum4 : Sum  OutDataTypeStr=single  SampleTime=2.08333333333333e-05  SaturateOnIntegerOverflow=on  InputSameDT=on
  Out1 : Outport
  wires:
  Sum4/1 -> Out1/1
  In2/1 -> Sum4/2
  In1/1 -> Sum4/1

== system AN_Simulink_Model_v1_fil/Auditory Nerve Model/Subsystem1/OHC LP Filter/Sum5 ==
  In1 : Inport
  In2 : Inport  Port=2
  Sum5 : Sum  OutDataTypeStr=single  SampleTime=2.08333333333333e-05  SaturateOnIntegerOverflow=on  InputSameDT=on
  Out1 : Outport
  wires:
  Sum5/1 -> Out1/1
  In2/1 -> Sum5/2
  In1/1 -> Sum5/1

== system AN_Simulink_Model_v1_fil/Auditory Nerve Model/Subsystem1/OHC LP Filter/Sum6 ==
  In1 : Inport
  In2 : Inport  Port=2
  Sum6 : Sum  OutDataTypeStr=single  SampleTime=2.08333333333333e-05  SaturateOnIntegerOverflow=on  InputSameDT=on
  Out1 : Outport
  wires:
  Sum6/1 -> Out1/1
  In2/1 -> Sum6/2
  In1/1 -> Sum6/1

== system AN_Simulink_Model_v1_fil/Auditory Nerve Model/Subsystem1/OHC LP Filter/Sum7 ==
  In1 : Inport
  In2 : Inport  Port=2
  Sum7 : Sum  OutDataTypeStr=single  SampleTime=2.08333333333333e-05  SaturateOnIntegerOverflow=on  InputSameDT=on
  Out1 : Outport
  wires:
  Sum7/1 -> Out1/1
  In2/1 -> Sum7/2
  In1/1 -> Sum7/1

== system AN_Simulink_Model_v1_fil/Auditory Nerve Model/Subsystem1/OHC NL Boltzman Function/Add1 ==
  In1 : Inport
  In2 : Inport  Port=2
  Add1 : Sum  OutDataTypeStr=single  SampleTime=2.08333333333333e-05  SaturateOnIntegerOverflow=on  InputSameDT=on
  Out1 : Outport
  wires:
  Add1/1 -> Out1/1
  In2/1 -> Add1/2
  In1/1 -> Add1/1

== system AN_Simulink_Model_v1_fil/Auditory Nerve Model/Subsystem1/OHC NL Boltzman Function/Add4 ==
  In1 : Inport
  In2 : Inport  Port=2
  Add4 : Sum  OutDataTypeStr=single  SampleTime=2.08333333333333e-05  SaturateOnIntegerOverflow=on  InputSameDT=on
  Out1 : Outport
  wires:
  Add4/1 -> Out1/1
  In2/1 -> Add4/2
  In1/1 -> Add4/1

== system AN_Simulink_Model_v1_fil/Auditory Nerve Model/Subsystem1/OHC NL Boltzman Function/Divide ==
  In1 : Inport
  In2 : Inport  Port=2
  Divide : Product  Inputs=*/  OutDataTypeStr=single  SampleTime=2.08333333333333e-05  SaturateOnIntegerOverflow=on  RndMeth=Zero
  Out1 : Outport
  wires:
  Divide/1 -> Out1/1
  In2/1 -> Divide/2
  In1/1 -> Divide/1

== system AN_Simulink_Model_v1_fil/Auditory Nerve Model/Subsystem1/OHC NL Boltzman Function/Divide1 ==
  In1 : Inport
  In2 : Inport  Port=2
  Divide1 : Product  Inputs=*/  OutDataTypeStr=single  SampleTime=2.08333333333333e-05  SaturateOnIntegerOverflow=on  RndMeth=Zero
  Out1 : Outport
  wires:
  Divide1/1 -> Out1/1
  In2/1 -> Divide1/2
  In1/1 -> Divide1/1

== system AN_Simulink_Model_v1_fil/Auditory Nerve Model/Subsystem1/OHC NL Boltzman Function/Divide2 ==
  In1 : Inport
  In2 : Inport  Port=2
  Divide2 : Product  Inputs=*/  OutDataTypeStr=single  SampleTime=2.08333333333333e-05  SaturateOnIntegerOverflow=on  RndMeth=Zero
  Out1 : Outport
  wires:
  Divide2/1 -> Out1/1
  In2/1 -> Divide2/2
  In1/1 -> Divide2/1

== system AN_Simulink_Model_v1_fil/Auditory Nerve Model/Subsystem1/OHC NL Boltzman Function/Divide3 ==
  In1 : Inport
  In2 : Inport  Port=2
  Divide3 : Product  Inputs=*/  OutDataTypeStr=single  SampleTime=2.08333333333333e-05  SaturateOnIntegerOverflow=on  RndMeth=Zero
  Out1 : Outport
  wires:
  Divide3/1 -> Out1/1
  In2/1 -> Divide3/2
  In1/1 -> Divide3/1

== system AN_Simulink_Model_v1_fil/Auditory Nerve Model/Subsystem1/OHC NL Boltzman Function/Gain1_unaryminus ==
  In1 : Inport
  Gain1_unaryminus : UnaryMinus  SampleTime=2.08333333333333e-05
  Out1 : Outport
  wires:
  Gain1_unaryminus/1 -> Out1/1
  In1/1 -> Gain1_unaryminus/1
